simulink model "EulerSolverTorque"  (R2016a)
settings: Solver=ode45  StartTime=0.0  StopTime=100.0  MaxStep=0.001  RelTol=1e-5  AbsTol=1e-5
values from neighbouring files (symbols this model uses):
  I = [3 3 7]    [EulerSolverTorque_Variables.m]
  w = [1 0 5]    [EulerSolverTorque_Variables.m]
settings Model: Creator=Kevin  LastModifiedBy=Kevin
settings GRTTargetCC: GeneratePreprocessorConditionals=Use local settings
settings SimscapeCC: SimscapeLogType=all  SimscapeLogDataHistory=10000

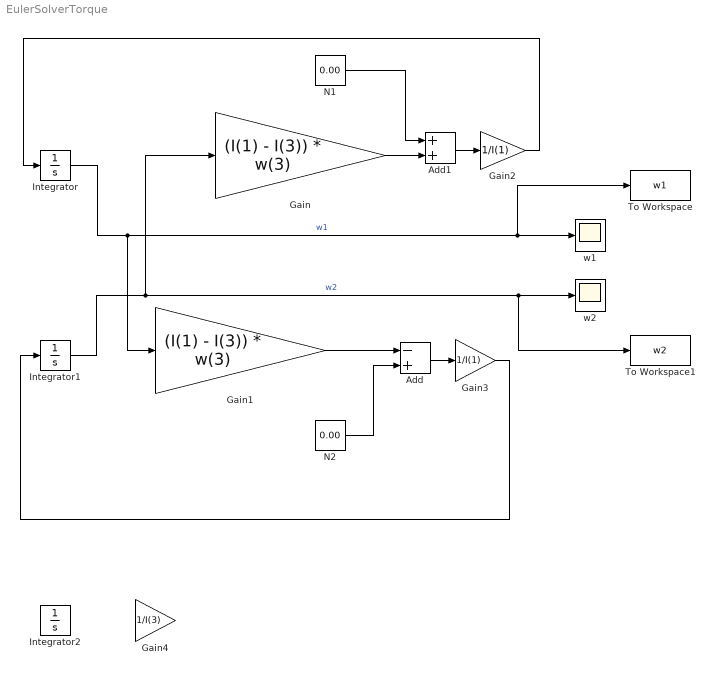
== system EulerSolverTorque ==
  Add : Sum  Inputs=-+
  Add1 : Sum
  Gain : Gain  Gain=(I(1) - I(3)) * w(3)
  Gain1 : Gain  Gain=(I(1) - I(3)) * w(3)
  Gain2 : Gain  Gain=1/I(1)
  Gain3 : Gain  Gain=1/I(1)
  Gain4 : Gain  Gain=1/I(3)
  Integrator : Integrator  InitialCondition=4
  Integrator1 : Integrator
  Integrator2 : Integrator
  N1 : Constant  Value=0.00
  N2 : Constant  Value=0.00
  To Workspace : ToWorkspace  VariableName=w1  SaveFormat=Timeseries  SampleTime=-1
  To Workspace1 : ToWorkspace  VariableName=w2  SaveFormat=Timeseries  SampleTime=-1
  w1 : Scope
  w2 : Scope
  wires:
  Gain2/1 -> Integrator/1
  Integrator/1 -> To Workspace/1, w1/1, Gain1/1  "w1"
  Integrator1/1 -> To Workspace1/1, w2/1, Gain/1  "w2"
  Gain1/1 -> Add/1
  Add1/1 -> Gain2/1
  Add/1 -> Gain3/1
  Gain3/1 -> Integrator1/1
  Gain/1 -> Add1/2
  N2/1 -> Add/2
  N1/1 -> Add1/1
